simulink model "OML58_Cores2"  (R2021b)
settings: Solver=ode1  StartTime=0.0  StopTime=10  FixedStep=Ts  RelTol=1e-3
PostLoadFcn:
  | Ts = 50e-6;
InitFcn:
  | Ts = 50e-6;
undefined symbols (not defined in the file): I, Left, Right, type, V, X
libraries: spsSeriesRLCBranchLib x30, artemis x20, spsThreePhaseSeriesRLCBranchLib x19, spsThreePhaseSeriesRLCLoadLib x15, spsThreePhaseBreakerLib x15, spsGroundLib x12, rtlab x9, LafaeLib x8, spsThreePhaseVIMeasurementLib x7, spsThreePhaseTransformerTwoWindingsLib x5, spsPower3phInstantaneousLib x5, spsStairGeneratorLib x2
(part 1 of 3)
settings Model: ARTEMISmethode_block_infos=$$__separator__$$OML58_Cores2/ARTEMIS Guide$$__separator__$$  Creator=LAFAE  LastModifiedBy=lafae
settings SolverCC: AlgebraicLoopSolver=TrustRegion
settings DataIOCC: ReturnWorkspaceOutputs=off
settings OptimizationCC: LocalBlockOutputs=off
settings DebuggingCC: SFMachineParentedDataDiag=warning  ArithmeticOperatorsInVariantConditions=warning
settings SFSimCC: CustomCodeUndefinedFunction=UseInterfaceOnly

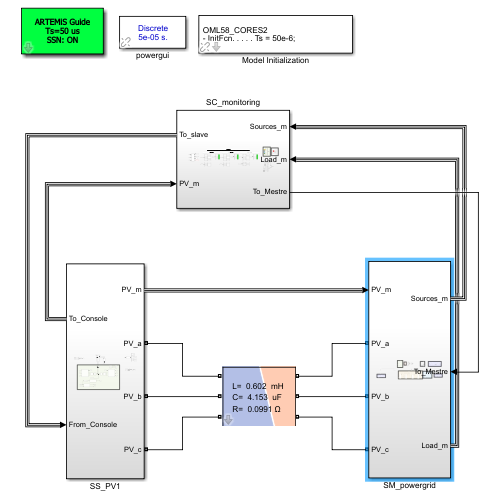
[thumbnail: Simulink's stored preview of the top-level diagram]
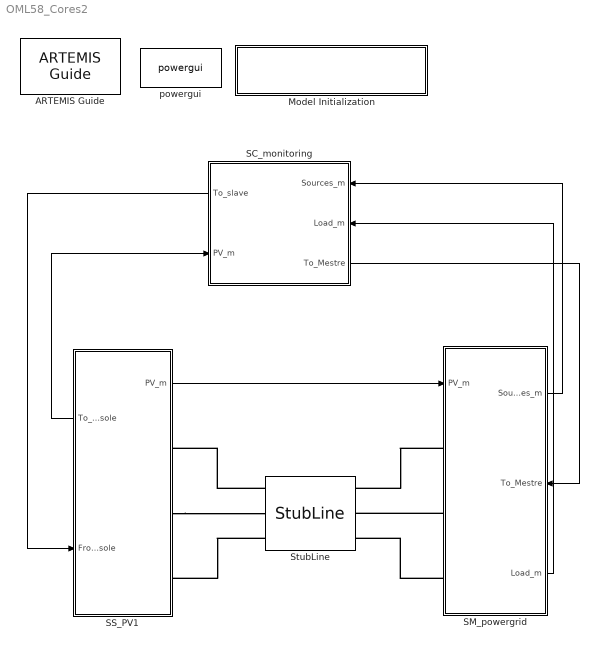
== system OML58_Cores2 ==
  ARTEMIS Guide : artemis/ARTEMIS/ARTEMIS Guide  Tag=art7.5  Description=New ARTEMiS block v 7.5b (R2015b+)  lock=on  Ts=Ts  ssn=on  opt=art5  dyna=off  nb_perm=4  RT_fullcomp=off  ssn_itvc=off  ssn_ivic=off  ssn_ext=off  ssn_solver=Art5 with Backward Euler nodal interface  iter_type=iSWITCH and iMOV only (default)  ssn_ImpulseLoopBlockedStateUpdate=5  ssn_mov_iter_number=5  ssn_switch_iter_number=3  ssn_lu_or_ldlt=LU (more robust)  ssn_nib_type_verify=off  ssn_use_lu=on  ssn_use_ldlt=off  ssn_impulse=on  ssn_quasimpulse=off  ssn_impulse_loop=5  paraExtinctionThy=off  Thy_Impulse=on  dtc=Off  dtc_opt=normal  ao=off  simtype=off  ct_mac=off  lin_mov=off  lsp=[0.001 2]  spike_skip=Disabled  dtc_extra=1  dtc_sws=normal  dtc_pied=0.5  SPSRulesBlock=SPSRules  tre=on  ctmm=off  LF=off  dpl_type=ARTEMiS DPL  rlc_type=off  custom_type=off  para=on  ssn_full_iteration=off  ssn_init_cond=block only
  Model Initialization : Subsystem  AncestorBlock=artemis/Tools /Misc/Model Initialization  mask(Model Functions){InitFcnX=Ts = 50e-6;, prel=off, posl=on, inif=on, strf=off}
      mask prompts: InitFcnX "Initialisation"; prel "Preload Function"; posl "PostLoad Function"; inif "InitFcn"; strf "StartFcn"
      mask init:
      | currentBlock = gcb;
      | root = bdroot(currentBlock);
      | 
      | if ~strcmp(get_param(root,'BlockDiagramType'),'library')
      |     if prel==1
      |         set_param(root, 'PreLoadFcn', InitFcnX);
      |     else
      |         set_param(root, 'PreLoadFcn', '');
      |     end
      |     if inif==1
      |         set_param(root, 'InitFcn', InitFcnX);
      |     else
      |         set_param(root, 'InitFcn', '');
      |     end
      |     if strf==1
      |         set_param(root, 'StartFcn', InitFcnX);
      |     else
      |         set_param(root, 'StartFcn', '');
      |     end
      |     if posl==1
      |         set_param(root, 'PostLoadFcn', InitFcnX);
      |     else
      |         set_param(root, 'PostLoadFcn', '');
      |     end
      | end
      | 
      | pos = get_param(currentBlock, 'Position');
      | width = pos(3) - pos(1); height = pos(4) - pos(2);
      | txt = [ upper(root) '\n' '- InitFcn. . . . . '  get_param(root, 'InitFcn') ];
      settings: CopyFcn=set_param(gcb,'LinkStatus','inactive')
      mask Display: text(5, height*0.5, txt, 'horizontalAlignment', 'left', 'verticalAlignment', 'middle') ;
  SC_monitoring : Subsystem
      settings: PortSchema="{\"entries\":[{\"content\":{\"sides\":[{\"content\":{\"connectorIds\":[\"Out2\",\"In1\"]},\"type\":\"ConnectorPlacement.EquallySpacedRectSide\",\"uuid\":\"12fdf98b-4c9f-4d37-8354-db891ff2ba57\"},{\"content\":{\"connectorIds\":[\"In2\",\"In3\",\"Out1\"],\"side\":\"RIGHT\"},\"type\":\"ConnectorPlacement.EquallySpacedRectSide\",\"uuid\":\"c8a60803-ac83-4983-9401-138bc9d7eb77\"},{\"content\":{\"connectorIds\":[],\"side\":\"TOP\"},\"type\":\"ConnectorPlacement.EquallySpacedRectSide\",\"uuid\":\"1621ea04-d943-45d1-951b-48cd31c23995\"},{\"content\":{\"connectorIds\":[],\"side\":\"BOTTOM\"},\"type\":\"ConnectorPlacement.EquallySpacedRectSide\",\"uuid\":\"b80cb71c-fbdc-4948-af33-fec5862caea8\"},{\"content\":{\"connectorIds\":[],\"side\":\"HIDDEN\"},\"type\":\"ConnectorPlacement.EquallySpacedRectSide\",\"uuid\":\"cabd082a-30d8-4f77-bd54-e7b85860f44b\"}]},\"type\":\"ConnectorPlacement.EquallySpacedConnector\",\"uuid\":\"f41e5cd0-195e-43de-9d9f-8b36e5f54d02\"}],\"packageUris\":[\"http://schema.mathworks.com/mf0/Connector/R2020b\"],\"version\":\"1.0\"}"
  SM_powergrid : Subsystem
      settings: PortSchema="{\"entries\":[{\"content\":{\"sides\":[{\"content\":{\"connectorIds\":[\"In1\",\"LConn1\",\"LConn2\",\"LConn3\"]},\"type\":\"ConnectorPlacement.EquallySpacedRectSide\",\"uuid\":\"04bb2d6e-c6da-4b85-8169-900f4989ab50\"},{\"content\":{\"connectorIds\":[\"Out1\",\"In2\",\"Out2\"],\"side\":\"RIGHT\"},\"type\":\"ConnectorPlacement.EquallySpacedRectSide\",\"uuid\":\"5f2c4f00-ae3e-4088-8f7b-f09f6f37f8dc\"},{\"content\":{\"connectorIds\":[],\"side\":\"TOP\"},\"type\":\"ConnectorPlacement.EquallySpacedRectSide\",\"uuid\":\"171dbadd-45da-46cb-b8b1-43862d1b9052\"}]},\"type\":\"ConnectorPlacement.EquallySpacedConnector\",\"uuid\":\"399874ae-d7cc-4980-ada2-ac9dc72741a6\"}],\"packageUris\":[\"http://schema.mathworks.com/mf0/Connector/R2020b\"],\"version\":\"1.0\"}"
  SS_PV1 : Subsystem
      settings: PortSchema="{\"entries\":[{\"content\":{\"sides\":[{\"content\":{\"connectorIds\":[\"Out2\",\"In1\"]},\"type\":\"ConnectorPlacement.EquallySpacedRectSide\",\"uuid\":\"c640b031-6784-4a25-a193-101771b28d9c\"},{\"content\":{\"connectorIds\":[\"Out1\",\"RConn1\",\"RConn2\",\"RConn3\"],\"side\":\"RIGHT\"},\"type\":\"ConnectorPlacement.EquallySpacedRectSide\",\"uuid\":\"6ef7a257-20e9-4181-b3e1-a43dc11aa4f4\"},{\"content\":{\"connectorIds\":[],\"side\":\"TOP\"},\"type\":\"ConnectorPlacement.EquallySpacedRectSide\",\"uuid\":\"b4b4a636-bb4e-4bbd-8626-98e203d7173d\"},{\"content\":{\"connectorIds\":[],\"side\":\"HIDDEN\"},\"type\":\"ConnectorPlacement.EquallySpacedRectSide\",\"uuid\":\"8c11410f-3f0b-408e-a3b2-4dee5c1b7994\"}]},\"type\":\"ConnectorPlacement.EquallySpacedConnector\",\"uuid\":\"0ec28515-f36e-4466-a6bd-24a57efcabb2\"}],\"packageUris\":[\"http://schema.mathworks.com/mf0/Connector/R2020b\"],\"version\":\"1.0\"}"
  StubLine : artemis/ARTEMIS/StubLine  Phases=3  pu=off  L=0.602e-3  Lpu=0.08  R=0.0991  Rpu=0.002  S_base=450e6/3  V_base=230e3/sqrt(3)  F_base=60  Ts=Ts
  powergui : spspowerguiLib/powergui  Priority=1  SimulationMode=Discrete  SampleTime=Ts  frequency=60  Iterations=50  frequencyindice=0  Pbase=100e6  ErrMax=1e-4  UnitsV=kV  UnitsW=MW  buscounter=0  FunctionMessages=off  echomessages=off  EnableUseOfTLC=off  CurrentSourceSwitches=off  DisableSnubberDevices=off  DisableRonSwitches=off  DisableVfSwitches=off  DisplayEquations=off  AutomaticDiscreteSolvers=off  SolverType=Tustin/Backward Euler (TBE)  Interpol=off  ExternalGateDelay=off  methode=off  Ts=100  x0status=blocks  SPID=on  SwTol=0  HookPort=off  NonlinearTolerance=1e-4  nMaxIteration=100  ContinueOnMaxIteration=off  RestoreLinks=warning  ResistiveCurrentMeasurement=off  Frange=[0:2:500]  Ylog=off  Xlog=on  ShowGrid=off  save=off  variable=ZData  structure=0  ZoomFFT=off  StartTime=0.0  cycles=1  DisplayStyle=1  fundamental=60  FreqAxis=off  MaxFrequency=1000  frequencyindicesteady=1  RmsSteady=1  display=off
  wires:
  SC_monitoring/2(To_slave) -> SS_PV1/1(From_Console)
  SS_PV1/1(PV_m) -> SM_powergrid/1(PV_m)
  SS_PV1/2(To_Console) -> SC_monitoring/1(PV_m)
  SM_powergrid/2(Load_m) -> SC_monitoring/3(Load_m)
  SM_powergrid/1(Sources_m) -> SC_monitoring/2(Sources_m)
  SC_monitoring/1(To_Mestre) -> SM_powergrid/2(To_Mestre)
  connections:
  SS_PV1/RConn2 -- StubLine/LConn2
  StubLine/LConn3 -- SS_PV1/RConn3
  StubLine/LConn1 -- SS_PV1/RConn1
  SM_powergrid/LConn2 -- StubLine/RConn2
  SM_powergrid/LConn1 -- StubLine/RConn1
  SM_powergrid/LConn3 -- StubLine/RConn3

== system OML58_Cores2/Model Initialization ==

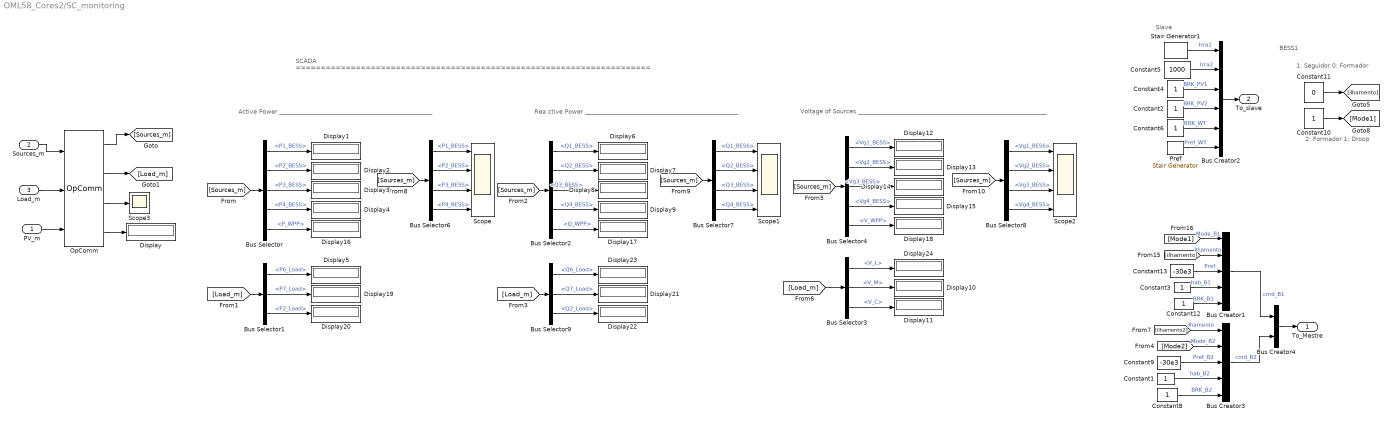
== system OML58_Cores2/SC_monitoring ==
  note: Slave
  note: BESS1
  note: 1: Seguidor
      | 0: Formador
  note: 2: Formador
      | 1: Droop
  note: SCADA
      | =======================================================================
  note: Rea ctive Power
      | ___________________________________________________
  note: Active Power
      | ___________________________________________________
  note: Voltage of Sources
      | _______________________________________________________________
  PV_m : Inport
  Sources_m : Inport  Port=2
  Load_m : Inport  Port=3
  Bus Creator1 : BusCreator  Inputs=5
  Bus Creator2 : BusCreator  Inputs=6
  Bus Creator3 : BusCreator  Inputs=5
  Bus Creator4 : BusCreator  Inputs=2
  Bus Selector : BusSelector  OutputSignals=BESS1.P1_BESS,BESS2.P2_BESS,BESS3.P3_BESS,BESS4.P4_BESS,WPP.P_WPP
  Bus Selector1 : BusSelector  OutputSignals=Load_L.P6_Load,Load_M.P7_Load,Load_C.P2_Load
  Bus Selector2 : BusSelector  OutputSignals=BESS1.Q1_BESS,BESS2.Q2_BESS,BESS3.Q3_BESS,BESS4.Q4_BESS,WPP.Q_WPP
  Bus Selector3 : BusSelector  OutputSignals=Load_L.V_L,Load_M.V_M,Load_C.V_C
  Bus Selector4 : BusSelector  OutputSignals=BESS1.Vg1_BESS,BESS2.Vg2_BESS,BESS3.Vg3_BESS,BESS4.Vg4_BESS,WPP.V_WPP
  Bus Selector6 : BusSelector  OutputSignals=BESS1.P1_BESS,BESS2.P2_BESS,BESS3.P3_BESS,BESS4.P4_BESS
  Bus Selector7 : BusSelector  OutputSignals=BESS1.Q1_BESS,BESS2.Q2_BESS,BESS3.Q3_BESS,BESS4.Q4_BESS
  Bus Selector8 : BusSelector  OutputSignals=BESS1.Vg1_BESS,BESS2.Vg2_BESS,BESS3.Vg3_BESS,BESS4.Vg4_BESS
  Bus Selector9 : BusSelector  OutputSignals=Load_L.Q6_Load,Load_M.Q7_Load,Load_C.Q2_Load
  Constant{1..4,6,8,10,12} (8 alike) : Constant
  Constant11 : Constant  Value=0
  Constant13 : Constant  Value=-30e3
  Constant5 : Constant  Value=1000
  Constant9 : Constant  Value=-30e3
  Display{,1..24} (25 alike) : Display
  OpComm : rtlab/OpComm  nbport=3  groupe_acq=1  subsys_rate=Ts  st=0  Synchronization=on  Interpolation=on  Threshold=1.0  Missed_Data=off  Sim_Time=on  Samples=off  dynSigOut=off  from_console=0  warning_done=off  writeOpCommFile=off  Offset=off
      settings: SourceProductName=RT-LAB
  Pref : spsStairGeneratorLib/Stair Generator  t=[0 4 7 9 12 16 25 35 47]  e=[1,0.7, 1, 1.0, 0, 0.7, 0.4, 0.2,1]  Ts=Ts
  Scope : Scope  NumInputPorts=4
  Scope1 : Scope  NumInputPorts=4
  Scope2 : Scope  NumInputPorts=4
  Scope3 : Scope
  Stair Generator1 : spsStairGeneratorLib/Stair Generator  t=[0, 1, 3, 5,7]  e=[10, 4, 7.5, 10,10]*1e2  Ts=0
  To_Mestre : Outport
  To_slave : Outport  Port=2
  wires:
  Stair Generator1/1 -> Bus Creator2/1  "Irra1"
  Constant5/1 -> Bus Creator2/2  "Irra2"
  Bus Creator2/1 -> To_slave/1
  Constant11/1 -> [ilhamento]
  Constant10/1 -> [Mode1]
  [Mode1] -> Bus Creator1/1  "Mode_B1"
  [ilhamento] -> Bus Creator1/2  "ilhamento"
  Constant13/1 -> Bus Creator1/3  "Pref"
  Constant3/1 -> Bus Creator1/4  "hab_B1"
  Constant12/1 -> Bus Creator1/5  "BRK_B1"
  [ilhamento2] -> Bus Creator3/1  "ilhamento"
  [Mode2] -> Bus Creator3/2  "Mode_B2"
  Constant9/1 -> Bus Creator3/3  "Pref_B2"
  Constant1/1 -> Bus Creator3/4  "hab_B2"
  Constant8/1 -> Bus Creator3/5  "BRK_B2"
  Bus Creator1/1 -> Bus Creator4/1  "cmd_B1"
  Bus Creator3/1 -> Bus Creator4/2  "cmd_B2"
  Constant4/1 -> Bus Creator2/3  "BRK_PV1"
  Constant2/1 -> Bus Creator2/4  "BRK_PV2"
  Constant6/1 -> Bus Creator2/5  "BRK_WT"
  Pref/1 -> Bus Creator2/6  "Pref_WT"
  OpComm/3 -> Scope3/1
  Bus Selector6/3 -> Scope/3  "<P3_BESS>"
  PV_m/1 -> OpComm/3
  [Load_m] -> Bus Selector9/1
  Bus Selector9/1 -> Display23/1  "<Q6_Load>"
  Bus Selector/4 -> Display4/1  "<P4_BESS>"
  Bus Selector7/1 -> Scope1/1  "<Q1_BESS>"
  Bus Selector/1 -> Display1/1  "<P1_BESS>"
  Bus Selector8/1 -> Scope2/1  "<Vg1_BESS>"
  Bus Selector8/4 -> Scope2/4  "<Vg4_BESS>"
  [Sources_m] -> Bus Selector2/1
  [Load_m] -> Bus Selector1/1
  Bus Selector4/3 -> Display14/1  "<Vg3_BESS>"
  Bus Selector7/3 -> Scope1/3  "<Q3_BESS>"
  Bus Selector8/3 -> Scope2/3  "<Vg3_BESS>"
  [Sources_m] -> Bus Selector7/1
  Bus Selector3/1 -> Display24/1  "<V_L>"
  Bus Selector9/2 -> Display21/1  "<Q7_Load>"
  Bus Selector4/5 -> Display18/1  "<V_WPP>"
  Bus Selector8/2 -> Scope2/2  "<Vg2_BESS>"
  Bus Selector6/1 -> Scope/1  "<P1_BESS>"
  Bus Selector2/5 -> Display17/1  "<Q_WPP>"
  Bus Selector1/3 -> Display20/1  "<P2_Load>"
  Bus Selector1/2 -> Display19/1  "<P7_Load>"
  [Sources_m] -> Bus Selector4/1
  OpComm/4 -> Display/1
  OpComm/2 -> [Load_m]
  Bus Selector3/2 -> Display10/1  "<V_M>"
  [Sources_m] -> Bus Selector/1
  [Sources_m] -> Bus Selector8/1
  Bus Selector7/2 -> Scope1/2  "<Q2_BESS>"
  Bus Selector6/4 -> Scope/4  "<P4_BESS>"
  Bus Selector/5 -> Display16/1  "<P_WPP>"
  Bus Selector/2 -> Display2/1  "<P2_BESS>"
  OpComm/1 -> [Sources_m]
  [Load_m] -> Bus Selector3/1
  Bus Selector9/3 -> Display22/1  "<Q2_Load>"
  Bus Selector4/4 -> Display15/1  "<Vg4_BESS>"
  Bus Selector1/1 -> Display5/1  "<P6_Load>"
  Bus Selector6/2 -> Scope/2  "<P2_BESS>"
  Bus Selector7/4 -> Scope1/4  "<Q4_BESS>"
  Bus Selector4/1 -> Display12/1  "<Vg1_BESS>"
  [Sources_m] -> Bus Selector6/1
  Load_m/1 -> OpComm/2
  Bus Selector3/3 -> Display11/1  "<V_C>"
  Bus Selector/3 -> Display3/1  "<P3_BESS>"
  Bus Selector2/4 -> Display9/1  "<Q4_BESS>"
  Sources_m/1 -> OpComm/1
  Bus Selector2/2 -> Display7/1  "<Q2_BESS>"
  Bus Selector4/2 -> Display13/1  "<Vg2_BESS>"
  Bus Selector2/1 -> Display6/1  "<Q1_BESS>"
  Bus Selector2/3 -> Display8/1  "<Q3_BESS>"
  Bus Creator4/1 -> To_Mestre/1
